simulink model "boat_controller"  (R2020a)
settings: Solver=FixedStepAuto  StartTime=0.0  StopTime=inf  RelTol=1e-3
PreLoadFcn:
  | % ROS setup
  | rosshutdown;
  | ipAddr = '';
  | rosinit(ipAddr)
  | 
  | % Sample times
  | sampleTime = 0.2;
  | 
  | % Control parameters
  | ctrlParam1 = 2;
  | ctrlParam2 = 3.5;
undefined symbols (not defined in the file or in its folder): controller, Rudder, sigbuilder_block, UBCSailbotBlocks, Winch
libraries: robotlib x4, simulink_extras x3, simulink x2
settings Model: Creator=scastro  LastModifiedBy=bruce
settings DataIOCC: ReturnWorkspaceOutputs=off
settings OptimizationCC: PassReuseOutputArgsAs=Individual arguments  MaxStackSize=64  EfficientTunableParamExpr=on
settings DebuggingCC: ParameterTunabilityLossMsg=error  ArithmeticOperatorsInVariantConditions=warning
settings HardwareCC: ProdBitPerLong=64  ProdHWDeviceType=Intel->x86-64 (Linux 64)
settings SFSimCC: SimUseLocalCustomCode=off  MATLABDynamicMemAlloc=off  CustomCodeUndefinedFunction=UseInterfaceOnly
settings RTWCC: SystemTargetFile=ert.tlc  HardwareBoard=Robot Operating System (ROS)  TemplateMakefile=ert_default_tmf  GenerateReport=on  RTWUseLocalCustomCode=off  Toolchain=Catkin  IncludeHyperlinkInReport=on  LaunchReport=on  PortableWordSizes=on  TargetLang=C++  GenerateTraceInfo=on  GenerateTraceReport=on  GenerateTraceReportSl=on  GenerateTraceReportSf=on  GenerateTraceReportEml=on
settings CodeAppCC: ForceParamTrailComments=on  IgnoreCustomStorageClasses=off  OperatorAnnotations=on  SimulinkDataObjDesc=on  SFDataObjDesc=on  InsertBlockDesc=on
settings ERTTargetCC: SupportContinuousTime=on  SupportVariableSizeSignals=on

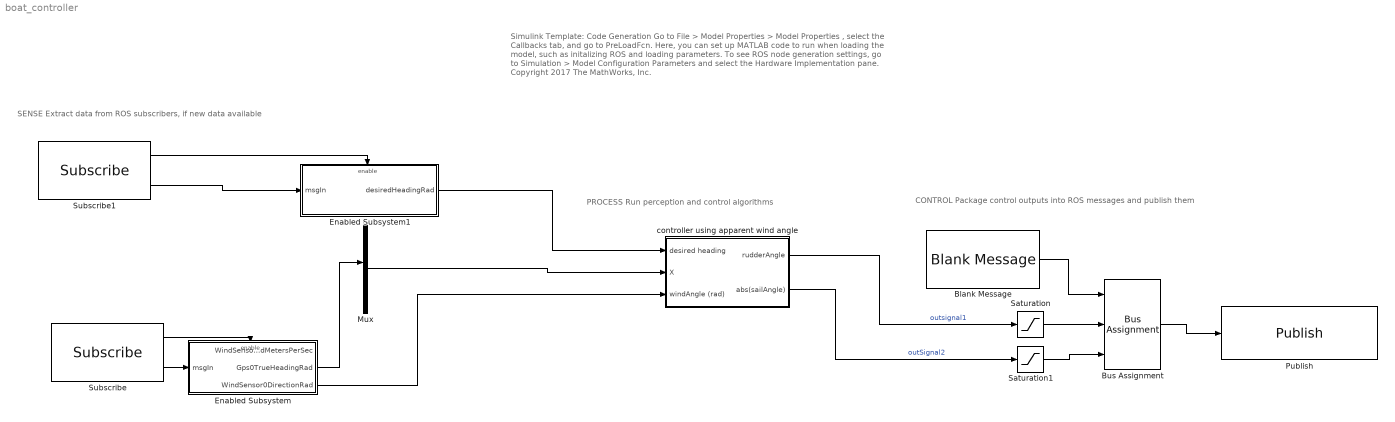
== system boat_controller ==
  note: PROCESS
      | Run perception and control algorithms
  note: SENSE
      | Extract data from ROS subscribers, if new data available
  note: CONTROL
      | Package control outputs into ROS messages and publish them
  note: Simulink Template: Code Generation
      |
      | Go to File > Model Properties > Model Properties , select the Callbacks tab, and go to PreLoadFcn. Here, you can set up MATLAB code to run when loading the model, such as initalizing ROS and loading parameters.
      |
      | To see ROS node generation settings, go to Simulation > Model Configuration Parameters and select the Hardware Implementation pane.
      |
      | Copyright 2017 The MathWorks, Inc.
  Blank Message : robotlib/Blank Message  messageClass=Message  entityType=sailbot_msg/actuation_angle  messageType=sailbot_msg/actuation_angle  SampleTime=inf
  Bus Assignment : BusAssignment  AssignedSignals=Rudder,Winch
  Enabled Subsystem : Subsystem  TreatAsAtomicUnit=on
  Enabled Subsystem1 : Subsystem  TreatAsAtomicUnit=on
  Mux : Mux  Inputs=8
  Publish : robotlib/Publish  topicSource=Specify your own  topic=/rudder_winch_actuation_angle  messageType=sailbot_msg/actuation_angle  messageQueueLength=1
  Saturation : Saturate  UpperLimit=pi/3  LowerLimit=-pi/3
  Saturation1 : Saturate  UpperLimit=pi/2  LowerLimit=0
  Subscribe : robotlib/Subscribe  topicSource=Specify your own  topic=/sensors  messageType=sailbot_msg/Sensors  sampleTime=-1  messageQueueLength=1
  Subscribe1 : robotlib/Subscribe  topicSource=Specify your own  topic=/heading  messageType=sailbot_msg/heading  sampleTime=-1  messageQueueLength=1
  controller using apparent wind angle : Subsystem  AncestorBlock=UBCSailbotBlocks/controller
  wires:
  Subscribe/2 -> Enabled Subsystem/1(msgIn)
  Subscribe/1 -> Enabled Subsystem/Enable
  Bus Assignment/1 -> Publish/1
  Blank Message/1 -> Bus Assignment/1
  controller using apparent wind angle/1(rudderAngle) -> Saturation/1  "outsignal1"
  controller using apparent wind angle/2(abs(sailAngle)) -> Saturation1/1  "outSignal2"
  Saturation/1 -> Bus Assignment/2
  Saturation1/1 -> Bus Assignment/3
  Enabled Subsystem/3(WindSensor0DirectionRad) -> controller using apparent wind angle/3(windAngle (rad))
  Mux/1 -> controller using apparent wind angle/2(X)
  Enabled Subsystem/2(Gps0TrueHeadingRad) -> Mux/4
  Subscribe1/1 -> Enabled Subsystem1/Enable
  Subscribe1/2 -> Enabled Subsystem1/1(msgIn)
  Enabled Subsystem1/1(desiredHeadingRad) -> controller using apparent wind angle/1(desired heading)

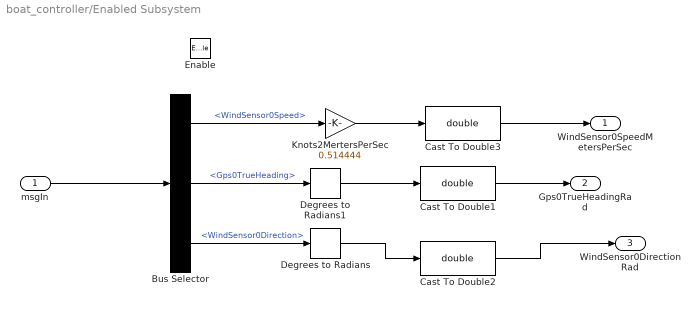
== system boat_controller/Enabled Subsystem ==
  msgIn : Inport
  Enable : EnablePort
  Bus Selector : BusSelector  OutputSignals=WindSensor0Speed,Gps0TrueHeading,WindSensor0Direction
  Cast To Double1 : DataTypeConversion  OutDataTypeStr=double
  Cast To Double2 : DataTypeConversion  OutDataTypeStr=double
  Cast To Double3 : DataTypeConversion  OutDataTypeStr=double
  Degrees to Radians : simulink_extras/Transformations/Degrees to Radians
  Degrees to Radians1 : simulink_extras/Transformations/Degrees to Radians
  Knots2MertersPerSec : Gain  Gain=0.514444
  WindSensor0SpeedMetersPerSec : Outport  VectorParamsAs1DForOutWhenUnconnected=off
  Gps0TrueHeadingRad : Outport  Port=2  VectorParamsAs1DForOutWhenUnconnected=off
  WindSensor0DirectionRad : Outport  Port=3  VectorParamsAs1DForOutWhenUnconnected=off
  wires:
  msgIn/1 -> Bus Selector/1
  Bus Selector/1 -> Knots2MertersPerSec/1  "<WindSensor0Speed>"
  Bus Selector/2 -> Degrees to Radians1/1  "<Gps0TrueHeading>"
  Bus Selector/3 -> Degrees to Radians/1  "<WindSensor0Direction>"
  Degrees to Radians1/1 -> Cast To Double1/1
  Knots2MertersPerSec/1 -> Cast To Double3/1
  Cast To Double1/1 -> Gps0TrueHeadingRad/1
  Cast To Double3/1 -> WindSensor0SpeedMetersPerSec/1
  Degrees to Radians/1 -> Cast To Double2/1
  Cast To Double2/1 -> WindSensor0DirectionRad/1

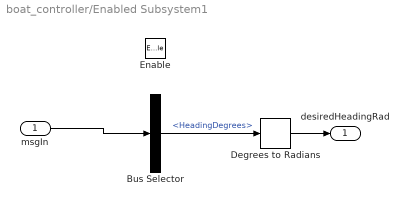
== system boat_controller/Enabled Subsystem1 ==
  msgIn : Inport
  Enable : EnablePort
  Bus Selector : BusSelector  OutputSignals=HeadingDegrees
  Degrees to Radians : simulink_extras/Transformations/Degrees to Radians
  desiredHeadingRad : Outport  VectorParamsAs1DForOutWhenUnconnected=off
  wires:
  msgIn/1 -> Bus Selector/1
  Bus Selector/1 -> Degrees to Radians/1  "<HeadingDegrees>"
  Degrees to Radians/1 -> desiredHeadingRad/1

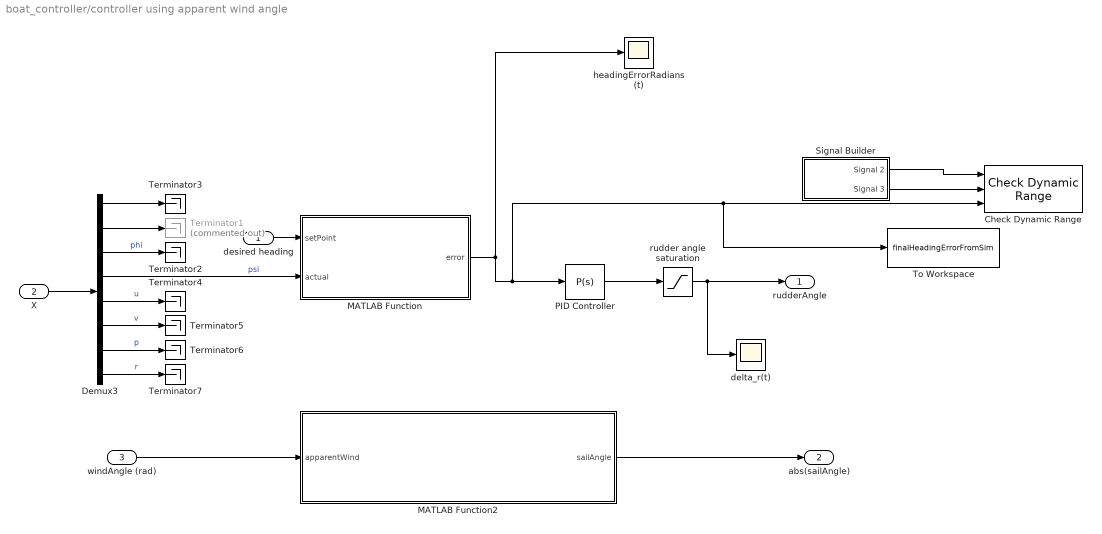
== system boat_controller/controller using apparent wind angle ==
  desired heading : Inport
  X : Inport  Port=2
  windAngle (rad) : Inport  Port=3
  Check Dynamic Range : simulink/Model Verification/Check  Dynamic Range  Description=min < u < max  enabled=off  stopWhenAssertionFail=on  export=off  icon=graphic
      settings: SourceProductBaseCode=SL
  Demux3 : Demux  Outputs=8
  MATLAB Function : MATLAB Function  TreatAsAtomicUnit=on
  MATLAB Function2 : MATLAB Function  TreatAsAtomicUnit=on
  PID Controller : simulink/Continuous/PID Controller  Controller=P  Form=Parallel  TimeDomain=Continuous-time  UseExternalTs=off  SampleTime=-1  IntegratorMethod=Forward Euler  FilterMethod=Forward Euler  ControllerParametersSource=internal  P=0.5  I=0  D=0  UseFilter=on  N=100  TunerSelectOption=Transfer Function Based (PID Tuner App)  InitialConditionSource=internal  InitialConditionForIntegrator=0  InitialConditionForFilter=0  DifferentiatorICPrevScaledInput=0  ExternalReset=none  TrackingMode=off  Kt=1  LimitOutput=off  UpperSaturationLimit=inf  LowerSaturationLimit=-inf  LinearizeAsGain=on  AntiWindupMode=none  Kb=1  POutMin=[]  POutMax=[]  IOutMin=[]  IOutMax=[]  DOutMin=[]  DOutMax=[]  NOutMin=[]  NOutMax=[]  SumOutMin=[]  SumOutMax=[]  SaturationOutMin=[]  SaturationOutMax=[]  PParamMin=[]  PParamMax=[]  IParamMin=[]  IParamMax=[]  DParamMin=[]  DParamMax=[]  NParamMin=[]  NParamMax=[]  KbParamMin=[]  KbParamMax=[]  KtParamMin=[]  KtParamMax=[]  KbOutMin=[]  KbOutMax=[]  KtOutMin=[]  KtOutMax=[]  IntegratorOutMin=[]  IntegratorOutMax=[]  FilterOutMin=[]  FilterOutMax=[]  SumI1OutMin=[]  SumI1OutMax=[]  SumI2OutMin=[]  SumI2OutMax=[]  SumI3OutMin=[]  SumI3OutMax=[]  SumI4OutMin=[]  SumI4OutMax=[]  SumDOutMin=[]  SumDOutMax=[]  DifferentiatorOutMin=[]  DifferentiatorOutMax=[]  FilterDiffOutCoefMin=[]  FilterDiffOutCoefMax=[]  ReciprocalOutMin=[]  ReciprocalOutMax=[]  SumDenOutMin=[]  SumDenOutMax=[]  SumNumOutMin=[]  SumNumOutMax=[]  DivideOutMin=[]  DivideOutMax=[]  UdiffTsProdOutMin=[]  UdiffTsProdOutMax=[]  NTsProdOutMin=[]  NTsProdOutMax=[]  UintegralTsProdOutMin=[]  UintegralTsProdOutMax=[]  UngainTsProdOutMin=[]  UngainTsProdOutMax=[]  IntegratorContinuousStateAttributes=''  IntegratorStateMustResolveToSignalObject=off  IntegratorRTWStateStorageClass=Auto  FilterContinuousStateAttributes=''  FilterStateMustResolveToSignalObject=off  FilterRTWStateStorageClass=Auto  ParallelPVariant=InternalParameters  IdealPVariant=Disabled  IVariant=Disabled  DVariant=Disabled  IntegratorVariant=Disabled  SatVariant=Disabled  AWVariant=Disabled  PCopyVariant=Disabled  TRVariant=Disabled  FdbkBlocksVariant=Forward  IdealPFdbkVariant=Disabled  SatFdbkVariant=Disabled  DerivativeFilterVariant=Disabled  NVariant=Disabled  NCopyVariant=Disabled_SignalSpec  FilterICVariant=Disabled  IntegratorICVariant=Disabled  ExternalResetVariant=Disabled  TRSumVariant=Passthrough  SumFdbkVariant=Disabled  SumVariant=Passthrough_P  TsampFilterVariant=InternalTs  TsampNgainVariant=Passthrough  TsampIntegralVariant=Disabled_SignalSpec
  Signal Builder : Subsystem  Tag=STV Subsys  LoadFcn=sigbuilder_block('load');  StartFcn=sigbuilder_block('start');  StopFcn=sigbuilder_block('stop');  ClipboardFcn=sigbuilder_block('clipboard');  mask(Sigbuilder block){tuvar=[0:10]}
      mask help: Simulink:masks:SigbuilderBlock_MD
      mask init:
      | if ~strcmp(get_param(bdroot(gcbh),'SimulationStatus'),'stopped') tuvar = sigbuilder_block('maskInit'); end
      settings: CopyFcn=sigbuilder_block('copy');  DeleteFcn=sigbuilder_block('delete');  ModelCloseFcn=sigbuilder_block('modelClose');  PreSaveFcn=sigbuilder_block('preSave');  PauseFcn=sigbuilder_block('pause');  ContinueFcn=sigbuilder_block('continue');  NameChangeFcn=sigbuilder_block('namechange');  OpenFcn=sigbuilder_block('open',[60 90 1141.5 522.75 ]);  CloseFcn=sigbuilder_block('close');
      mask Display: plot(0, 0, 100, 100,[2, 2, 32, 32, 2], [68, 8, 8, 68, 68],[32, 2], [38, 38], [32, 19, 2],[53, 60, 44], [32, 17, 17, 2],[16, 16, 31, 31]);txt = getActiveGroup(gcbh);text(2, 100, txt,'verticalAlignment', 'top');
  Terminator1 : Terminator  Commented=on
  Terminator{2..7} (6 alike) : Terminator
  To Workspace : ToWorkspace  VariableName=finalHeadingErrorFromSim  SampleTime=-1
      settings: MaxDataPoints=1  Save2DSignal=2-D array (concatenate along first dimension)
  delta_r(t) : Scope
  headingErrorRadians (t) : Scope
  rudder angle saturation : Saturate  UpperLimit=pi/3  LowerLimit=-pi/3  LinearizeAsGain=off
  rudderAngle : Outport
  abs(sailAngle) : Outport  Port=2
  wires:
  MATLAB Function2/1(sailAngle) -> abs(sailAngle)/1
  windAngle (rad)/1 -> MATLAB Function2/1(apparentWind)
  PID Controller/1 -> rudder angle saturation/1
  MATLAB Function/1(error) -> headingErrorRadians (t)/1, PID Controller/1, Check Dynamic Range/3, To Workspace/1
  rudder angle saturation/1 -> rudderAngle/1, delta_r(t)/1
  Signal Builder/2(Signal 3) -> Check Dynamic Range/2
  Signal Builder/1(Signal 2) -> Check Dynamic Range/1
  desired heading/1 -> MATLAB Function/1(setPoint)
  Demux3/8 -> Terminator7/1  "r"
  Demux3/7 -> Terminator6/1  "p"
  Demux3/6 -> Terminator5/1  "v"
  Demux3/5 -> Terminator4/1  "u"
  Demux3/3 -> Terminator2/1  "phi"
  Demux3/2 -> Terminator1/1
  Demux3/1 -> Terminator3/1
  X/1 -> Demux3/1
  Demux3/4 -> MATLAB Function/2(actual)  "psi"

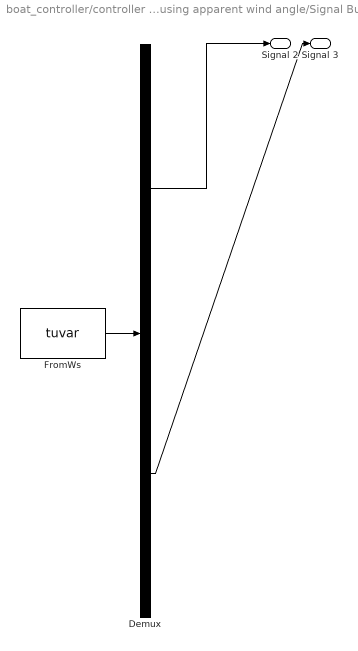
== system boat_controller/controller using apparent wind angle/Signal Builder ==
  Demux : Demux  Tag=STV Demux  Outputs=2
      settings: DisplayOption=none
  FromWs : FromWorkspace  Tag=STV FromWs  VariableName=tuvar
      SigBuilderData=|
      | common.afterFinalStr = 'Extrapolate'
      | common.sampleTime = 0
      | dataSet.timeRange = [0 100]
      | dataSet.name = 'Group 1'
      | sbobj.Groups.Name = 'Group 1'
      | sbobj.Groups.Signals(1).Name = 'Signal 2'
      | sbobj.Groups.Signals(1).XData = [0 50 50 60 100]
      | sbobj.Groups.Signals(1).YData = [100 100 0.3 0.2 0.2]
      | sbobj.Groups.Signals(2).Name = 'Signal 3'
      | sbobj.Groups.Signals(2).XData = [0 50 50 60 100]
      | sbobj.Groups.Signals(2).YData = [-100 -100 -0.3 -0.2 -0.2]
      | sbobj.Groups.TimeRange = [0 100]
  Signal 2 : Outport  Tag=STV Outport
  Signal 3 : Outport  Tag=STV Outport  Port=2
  wires:
  Demux/2 -> Signal 3/1
  Demux/1 -> Signal 2/1
  FromWs/1 -> Demux/1

== matlab function boat_controller/controller using apparent wind angle/MATLAB Function ==
  data: setPoint input; error output; actual input
function error = getHeadingError(setPoint,actual)
error = getHeadingError(setPoint,actual);
end

== matlab function boat_controller/controller using apparent wind angle/MATLAB Function2 ==
  data: apparentWind input; sailAngle output
function sailAngle = getSailAngleWrapper(apparentWind)

sailAngle = getSailAngle(apparentWind);
